simulink model "model"  (Simulink 7.7)
settings: Solver=ode45  StartTime=0.0  StopTime=100.0  RelTol=1e-3
settings Model: Creator=Jakub  LastModifiedBy=Jakub

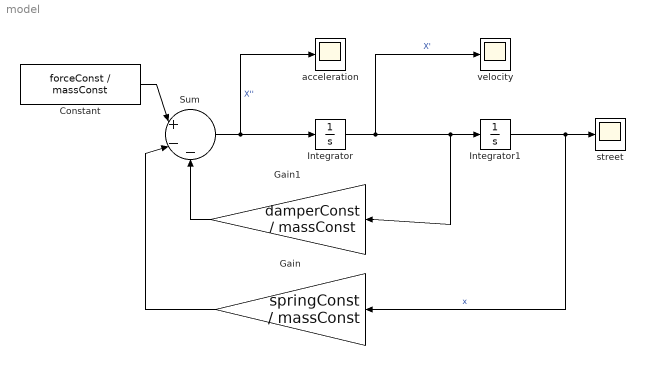
== system model ==
  Constant : Constant  Value=forceConst / massConst
  Gain : Gain  Gain=springConst / massConst
  Gain1 : Gain  Gain=damperConst / massConst
  Integrator : Integrator
  Integrator1 : Integrator
  Sum : Sum  Inputs=|+--
  acceleration : Scope
  street : Scope
      settings: SaveName=ScopeData2
  velocity : Scope
  wires:
  Integrator/1 -> velocity/1, Integrator1/1, Gain1/1  "X'"
  Integrator1/1 -> street/1, Gain/1  "x"
  Sum/1 -> Integrator/1, acceleration/1  "X''"
  Constant/1 -> Sum/1
  Gain1/1 -> Sum/3
  Gain/1 -> Sum/2
